simulink model "KF_POC_sim"  (R2018a)
settings: Solver=VariableStepAuto  StartTime=0.0  StopTime=10.0  RelTol=1e-3
settings Model: Creator=hammane  LastModifiedBy=hammane

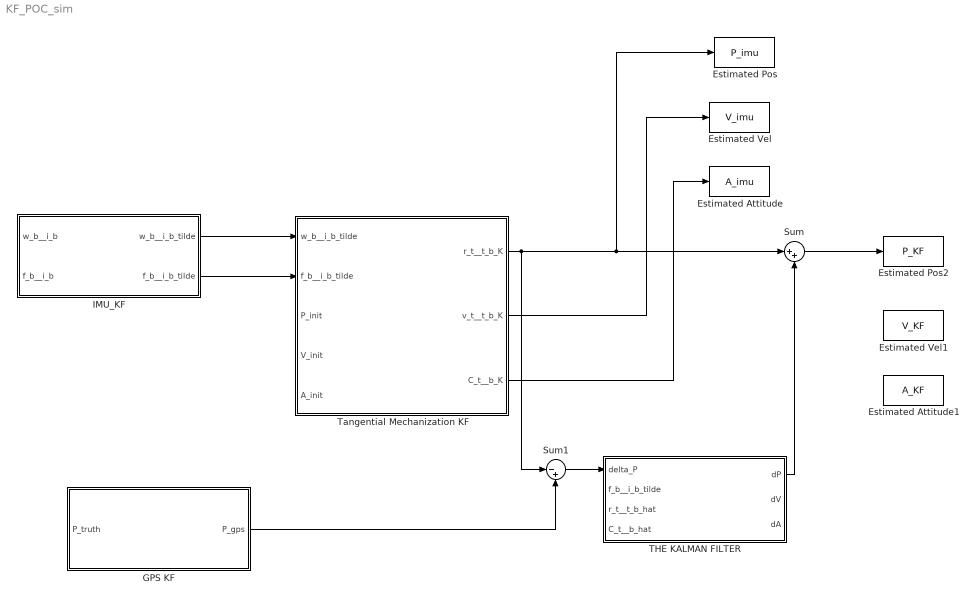
== system KF_POC_sim ==
  Estimated Attitude : ToWorkspace  VariableName=A_imu  SampleTime=-1
  Estimated Attitude1 : ToWorkspace  VariableName=A_KF  SampleTime=-1
  Estimated Pos : ToWorkspace  VariableName=P_imu  SampleTime=-1
  Estimated Pos2 : ToWorkspace  VariableName=P_KF  SampleTime=-1
  Estimated Vel : ToWorkspace  VariableName=V_imu  SampleTime=-1
  Estimated Vel1 : ToWorkspace  VariableName=V_KF  SampleTime=-1
  GPS KF : MATLAB Function  TreatAsAtomicUnit=on
  IMU_KF : MATLAB Function  TreatAsAtomicUnit=on
  Sum : Sum  Inputs=|++
  Sum1 : Sum  Inputs=|-+
  THE KALMAN FILTER : MATLAB Function  TreatAsAtomicUnit=on
  Tangential Mechanization KF : MATLAB Function  TreatAsAtomicUnit=on
  wires:
  Tangential Mechanization KF/1(r_t__t_b_K) -> Sum1/1, Sum/1, Estimated Pos/1
  Tangential Mechanization KF/2(v_t__t_b_K) -> Estimated Vel/1
  Tangential Mechanization KF/3(C_t__b_K) -> Estimated Attitude/1
  THE KALMAN FILTER/1(dP) -> Sum/2
  Sum/1 -> Estimated Pos2/1
  GPS KF/1(P_gps) -> Sum1/2
  Sum1/1 -> THE KALMAN FILTER/1(delta_P)
  IMU_KF/1(w_b__i_b_tilde) -> Tangential Mechanization KF/1(w_b__i_b_tilde)
  IMU_KF/2(f_b__i_b_tilde) -> Tangential Mechanization KF/2(f_b__i_b_tilde)

== matlab function KF_POC_sim/IMU_KF ==
  data: w_b__i_b input; f_b__i_b input; constants parameter; w_b__i_b_tilde output; f_b__i_b_tilde output
function [w_b__i_b_tilde, f_b__i_b_tilde] = IMU_KF(w_b__i_b, f_b__i_b, constants)
%#codegen
% FUNCTION DESCRIPTION:
%   Simulation of an IMU (ideal error-free case)
%
% INPUTS:
%   w_i__i_b = Angular velocity of {b} wrt {i} resolved in {i} (rad/s)
%   a_i__i_b = Acceleration     of {b} wrt {i} resolved in {i} (m/s^2)
%   constants= A structure containing many constant parameters
%
% OUTPUTS:
%   w_b__i_b_tilde = Gyro  meas (rad/s)
%   f_b__i_b_tilde = Accel meas (m/s^2)
%
% NOTES:
%   - None
%
% REFERENCE:
%   http://mercury.pr.erau.edu/~bruders EE 440 Modern Navigation

persistent b_g_BI b_a_BI                            % Persistent storage class variables

if isempty(b_g_BI)
    b_g_BI       = [0; 0; 0];                       % Initialize the Markov Bias Instability Bias term (rad/s)
    b_a_BI       = [0; 0; 0];                       % Initialize the Markov Bias Instability Bias term (m/s^2)     
end

dt           = constants.dt;    % Time step
I3           = eye(3);          % Identity matrix
Fs           = constants.Fs;    % Sample frequency
 % Gyro  related terms   
b_g_BI_sigma_n = constants.gyro.BI.sigma_n;         % Bias - White noise driving the Bias Instability 1-sigma (rad/s)

tau_g        = constants.gyro.BI.correlation_time;  % Correlation time for the bias instability (sec)
b_g_FB       = constants.gyro.b_g_FB;               % Bias - Fixed Bias term (rad/s)

sigma_ARW   = constants.gyro.sigma_ARW;             % Standard deviation of white noise due to ARW (rad/s)
M_g         = constants.gyro.M_g;                   % The combined Gyro Misalignment/Scale-Factor matrix
G_g         = constants.gyro.G_g;                   % The gyro G-sensitivity matrix (rad/sec/g)

 % Accel related terms   
b_a_BI_sigma_n = constants.accel.BI.sigma_n;        % Bias - White noise driving the Bias Instability 1-sigma (m/s^2)

tau_a        = constants.accel.BI.correlation_time; % Correlation time for the bias instability (sec)
b_a_FB       = constants.accel.b_a_FB;              % Bias - Fixed Bias term (m/s^2)

sigma_VRW   = constants.accel.sigma_VRW;            % Standard deviation of white noise due to VRW (m/s^2)
M_a         = constants.accel.M_a;                  % The combined Gyro Misalignment/Scale-Factor matrix    

%++++++++++++++++++++++++++++++++++++++++++++++++++++++++++++++++++++++++++
% Gyro Model:
%++++++++++++++++++++++++++++++++++++++++++++++++++++++++++++++++++++++++++

% Bias terms
b_g_BS = constants.gyro.b_g_BS;             % Bias - Bias Stability Bias term (rad/s)
b_g_BI = exp(-dt/tau_g) * b_g_BI + randn(3,1)*b_g_BI_sigma_n; % Bias - Markov Bias Instability Bias term (rad/s)
b_g = b_g_BI + b_g_FB + b_g_BS;             % All three bias terms (rad/s)

% Noise terms
w_g = sigma_ARW * randn(3,1);        % Gyro noise (rad/sec)

% Including all of the error terms
w_b__i_b_tilde = b_g + (I3 + M_g) * w_b__i_b + G_g * f_b__i_b + w_g;

%++++++++++++++++++++++++++++++++++++++++++++++++++++++++++++++++++++++++++
% Accelerometer Model
%++++++++++++++++++++++++++++++++++++++++++++++++++++++++++++++++++++++++++

% Bias terms
b_a_BS = constants.accel.b_a_BS;             % Bias - Bias Stability Bias term (m/s^2)
b_a_BI = exp(-dt/tau_a) * b_a_BI + randn(3,1)*b_a_BI_sigma_n; % Bias - Markov Bias Instability Bias term (m/s^2)
b_a = b_a_BI + b_a_FB + b_a_BS;             % All three bias terms (m/s^2)

% Noise terms
w_a = sigma_VRW * randn(3,1);        % Accelerometer noise (in m/s^2)

% Including all of the error terms
f_b__i_b_tilde = b_a + (I3 + M_a) * f_b__i_b + w_a;

== matlab function KF_POC_sim/Tangential Mechanization KF ==
  data: w_b__i_b_tilde input; r_t__t_b_K output; f_b__i_b_tilde input; P_init input; V_init input; A_init input; constants parameter; v_t__t_b_K output; C_t__b_K output
function [r_t__t_b_K, v_t__t_b_K, C_t__b_K] = TAN_mech_KF(w_b__i_b_tilde, f_b__i_b_tilde, P_init, V_init, A_init, constants)
%#codegen
% FUNCTION DESCRIPTION:
%   Implements the low and high-fidelity Tangential Frame Mechanization
%
% INPUTS:
%   w_b__i_b_tilde  = Current Gyro measurements (rad/s)
%   f_b__i_b_tilde  = Current Accel measurements (m/s^2)
%   P_init          = True position r_t__t_b used to initialize (meters)
%   V_init          = True velocity v_t__t_b used to initialize (meters/sec)
%   A_init          = True attitude C_t__b used to initialize (dimless)
%
% OUTPUTS:
%   r_t__t_b_K      = Updated position r_t__t_b(k) = r_t__t_b(+) (meters)
%   v_t__t_b_K      = Updated velocity v_t__t_b(k) = v_t__t_b(+) (meters/sec)
%   C_t__b_K        = Updated attitude C_t__b(k)   = C_t__b(+)
%
%  Reference:  EE 440 Lecture notes:
%
%  NOTES:
%   1.) fidelity = 0 => Low-fidelity or = 1 => High-fidelity
%   2.) The True PVA is ONLY used to initialize the mechanization!!

persistent r_t__t_b_K_1 v_t__t_b_K_1 C_t__b_K_1

fidelity = constants.fidelity;      % Set to '0' for Low-fidelity and '1' for High-fidelity
dt       = constants.dt;            % Time step (sec)
I3       = eye(3);                  % 3X3 Identity matrix
Ohm_i__i_e = constants.Ohm_i__i_e;  % Earth Rate skew-symmetric matrix (rad/s)
w_i__i_e   = constants.w_i__i_e;    % Angular velocity of {e} wrt {i} resolved in {i} (rad/s)
C_e__t = constants.C_e__t;          % Attitude of t-frame wrt e-frame (a constant matrix)
C_t__e = C_e__t';
r_e__e_t = constants.r_e__e_t;      % Position of org of t-frame wrt e-frame resolved in e-frame

% If this is the first call to the function then Initialize the PVA
if isempty(C_t__b_K_1)      % Initialize the PVA (with zero for everything)
    r_t__t_b_K = P_init;
    v_t__t_b_K = V_init;
    C_t__b_K   = A_init;
    
    % Update PVA(k-1) = PVA(-) values
    r_t__t_b_K_1 = P_init; % Body and nav frame share common org
    v_t__t_b_K_1 = V_init;
    C_t__b_K_1   = A_init;
else
%==========================================================================
% Tangential Frame PVA Mechanization:
%==========================================================================
    Ohm_t__i_e = C_t__e * Ohm_i__i_e * C_e__t; % Earth rate in the t-frame
    
    %----------------------------------------------------------------------
    % STEP 1.) Attitude Update
    %----------------------------------------------------------------------    
    if ~fidelity                    % If "low-fidelity" eqns

    % First order approximation used (Lower fidelity eqns) ++++++++++++++++++++
    % Build skew-symmetric matrix Ohm from vector w
    Ohm_b__i_b_tilde = vec2ss(w_b__i_b_tilde); % (rad/s)
    %  t       t              b             t    t
    % C (k) = C (k-1) [I + Ohm (k) dt] - Ohm    C (k-1)
    %  b       b              ib            ie   b
    C_t__b_K = C_t__b_K_1 * (I3 + Ohm_b__i_b_tilde*dt) - Ohm_t__i_e * C_t__b_K_1*dt;

    else                            % If "high-fidelity" eqns
    % Higher fidelity equations +++++++++++++++++++++++++++++++++++++++++++++++
    %   t        t  b        t
    %  w  (k) = C  w  (k) - w 
    %   tb       b  ib       ie
    w_t__t_b = C_t__b_K_1 * w_b__i_b_tilde - C_t__e * w_i__i_e;  % (rad/s)
    %            t
    % Defining: w   dt = k d_theta, and K = Skew(k)
    %            tb
    
    %  t                                               2     t
    % C (k) = [I + sin(d_theta) K + (1 - cos(d_theta) K )]  C (k-1) 
    %  b                                                     b
    %
    C_t__b_K = Rodrigues_k(w_t__t_b*dt) * C_t__b_K_1; % 
    end
    
    %--------------------------------------------------------------------------
    % STEP 2.) Specific Force Update
    %----------------------------------------------------------------------
    %  t     t     b  
    % f   = C (k) f
    %  ib    b     ib
    f_t__i_b = C_t__b_K * f_b__i_b_tilde;   % (m/s^2)

    %--------------------------------------------------------------------------
    % STEP 3.) Velocity Update
    %----------------------------------------------------------------------
    % Gravity Calculation:
    % Since the body is above the ellipsoid use the "gravity" fn NOT Somigliana
    r_e__e_b = r_e__e_t + C_e__t * r_t__t_b_K_1;            % Compute r_e__e_b
    [L_b, lambda_b, h_b] = xyz2llh(r_e__e_b, constants);    % Compute the lat, lon, and height
    g_n__b = [0; 0; gravity(L_b, h_b, constants)];          % Compute the acceleration due to gravity
    C_e__n = Lat_Lon_2C_e__n(L_b, lambda_b);                % Compute C_e__n
    g_e__b = C_e__n * g_n__b;                               % Compute the gravity of the body in the {e} frame
    g_t__b = C_t__e * g_e__b;                               % Compute the gravity of the body in the {t} frame
    
    %  t    t     t        t   t
    % a  = f   + g  - 2 Ohm   v  (k-1)
    %  tb   ib    b        ie  tb
    a_t__t_b = f_t__i_b + g_t__b - 2*Ohm_t__i_e * v_t__t_b_K_1; % (m/s^2)

    %   t        t          t
    %  v  (k) = v  (k-1) + a   dt
    %   tb       tb         tb
    v_t__t_b_K = v_t__t_b_K_1 + a_t__t_b * dt;  % (m/s)

    %--------------------------------------------------------------------------
    % STEP 4.) Position Update
    %----------------------------------------------------------------------
    %   t        t          t             t         2
    %  r  (k) = r  (k-1) + v  (k-1) dt + a  (k-1) dt
    %   tb       tb         tb            tb
    r_t__t_b_K = r_t__t_b_K_1 + v_t__t_b_K_1*dt + a_t__t_b * dt^2 / 2; % slide 8 (m)
    
    % Store PVA(k-1) values for use in next iteration
    r_t__t_b_K_1 = r_t__t_b_K; % Body and nav frame share common org
    v_t__t_b_K_1 = v_t__t_b_K;
    C_t__b_K_1   = C_t__b_K;
end  % End of the t_sec == 0 block

end     % End of function

== matlab function KF_POC_sim/GPS KF ==
  data: P_truth input; constants parameter; P_gps output
function P_gps  = GPS_KF(P_truth, constants)
%#codegen
% FUNCTION DESCRIPTION:
%   Simulation of an IMU (ideal error-free case)
%
% INPUTS:
%   w_i__i_b = Angular velocity of {b} wrt {i} resolved in {i} (rad/s)
%   a_i__i_b = Acceleration     of {b} wrt {i} resolved in {i} (m/s^2)
%   constants= A structure containing many constant parameters
%
% OUTPUTS:
%   w_b__i_b_tilde = Gyro  meas (rad/s)
%   f_b__i_b_tilde = Accel meas (m/s^2)
%
% NOTES:
%   - None
%
% REFERENCE:
%   http://mercury.pr.erau.edu/~bruders EE 440 Modern Navigation
% Take truth data and expand to measured GPS data

    sigma = constants.gps.sigma;                            % Radius of error
    P_error = normrnd(0,sigma,3,1);                % Error = radius of error * rand value
    P_gps = P_truth + P_error;                      % GPS = Truth + Error 
end

== matlab function KF_POC_sim/THE KALMAN FILTER ==
  data: delta_P input; f_b__i_b_tilde input; r_t__t_b_hat input; C_t__b_hat input; constants parameter; dP output; dV output; dA output
function [dP, dV, dA] = The_Kalman(delta_P, f_b__i_b_tilde, r_t__t_b_hat, C_t__b_hat, constants)
I3 = eye(3);
O3 = zeros(3);
sigma_gps = constants.gps.sigma;
dt         = constants.dt;          % Time step (sec)
Ohm_i__i_e = constants.Ohm_i__i_e;  % Skew symmetric version of w_i__i_e (rad/s)
C_e__t     = constants.C_e__t;   	% Attitude of t-frame wrt e-frame (a constant matrix)
C_t__e     = C_e__t';
r_e__e_t   = constants.r_e__e_t;    % Position of org of t-frame wrt e-frame resolved in e-frame
Df_b__i_b = constants.accel.BI.sigma_n;     % Assume error in accel is all BI
Dw_b__i_b = constants.gyro.BI.sigma_n;      % Assume error in gyro is all BI

persistent Delta_PVAk_1 P_k_1
   
if isempty(Delta_PVAk_1)    
    Delta_PVAk_1  = zeros(9,1);     % Initialize Delta_PVA(k-1)
    Delta_PVAk    = zeros(9,1);     % Initialize Delta_PVA(k-1)
    P_k_1         = 0.1 * eye(9);
    P_k           = 0.1 * eye(9);
else
%% Build the F matrix: See lecture 29 slide 7
    O3 = zeros(3,3);
% First row:
    Ohm_t__i_e = C_t__e * Ohm_i__i_e * C_e__t;  % Earth rate in the t-frame

% Second row:
    F21 = -vec2ss(C_t__b_hat * f_b__i_b_tilde); % Vector to Skew-Symmetric
  % Now build F23
    r_e__e_b_hat = r_e__e_t + C_e__t * r_t__t_b_hat;
    [L_b_hat, lambda_b_hat, h_b_hat] = xyz2llh(r_e__e_b_hat, constants);
    gamma_e__i_b = gamma__i_b(r_e__e_b_hat, constants);
    r_e__e_S = Geo_Radius(L_b_hat, constants);
 
    F23 = -C_t__e * 2 * gamma_e__i_b * r_e__e_b_hat' / (r_e__e_S * norm(r_e__e_b_hat)) * C_e__t;
     
    F = [ -Ohm_t__i_e   ,  O3               , O3
           F21          , -2* Ohm_t__i_e    , F23
           O3           ,  I3               , O3];

%% Build the B matrix: See lecture 29 slide 7
    B = [C_t__b_hat * Dw_b__i_b
         C_t__b_hat * Df_b__i_b
         O3];
%% Transform Eqns from continuous-time to discrete-time: Lecture 30 slides 9-10
    A = eye(9) + F*dt;                % Estimate of exp(F dt) = I + F dt + F^2 dt^2 /2! + ...
	Q = eye(9)*0.01;
    G  = (eye(9)*dt + F*dt^2/2) * B;    % Estimate of G = A^-1 (exp(F dt) - I ) B = (I dt + F dt^2 /2! + ...) B
    
    H = [I3, O3, O3];                   % Only have delta Position
    R = I3*sigma_gps;                       % R is based on the sigma of GPS
    [Delta_PVAk, P_k] = Kalman_Filter(Delta_PVAk_1, P_k_1, delta_P, A, H, Q, R, O3, O3);

    Delta_PVAk_1 = Delta_PVAk;
    P_k_1 = P_k;
end

    dP = Delta_PVAk(1:3,1);
    dV = Delta_PVAk(4:6,1);
    dA = Delta_PVAk(7:9,1);


end     % End of function
